simulink model "reaktor"  (R2016a)
settings: Solver=VariableStepAuto  StartTime=0.0  StopTime=300  RelTol=1e-3
values from neighbouring files (symbols this model uses):
  B = 0.0064    [Unit_3.m]    (also in reactor_pocz.m; unit_1.m; unit_4.m)
  C_psi = 13.75 * (10 ^ 6)    (= 13750000)    [Unit_3.m]    (also in reactor_pocz.m; unit_4.m)
  LAMBDA = 10 ^ -5    (= 1e-05)    [Unit_3.m]    (also in reactor_pocz.m; unit_1.m; unit_4.m)
  lambda = 0.1    [Unit_3.m]    (also in reactor_pocz.m; unit_1.m; unit_4.m)
  P_1 = -1.223 * (10 ^ -4)    (= -0.0001223)    [Unit_3.m]    (also in reactor_pocz.m; unit_1.m = -0.0001322; unit_4.m = -0.0001286)
  P_2 = -5.502 * (10 ^ -5)    (= -5.502e-05)    [Unit_3.m]    (also in reactor_pocz.m; unit_1.m = -6.08e-05; unit_4.m = -6.79e-05)
  P_3 = -1.953 * (10 ^ -4)    (= -0.0001953)    [Unit_3.m]    (also in reactor_pocz.m; unit_1.m = -0.000285; unit_4.m = -0.0002887)
  S = 1938.9    [Unit_3.m]    (also in reactor_pocz.m; unit_1.m = 2859; unit_4.m = 2910.3)
settings Model: Creator=Użytkownik  LastModifiedBy=Użytkownik

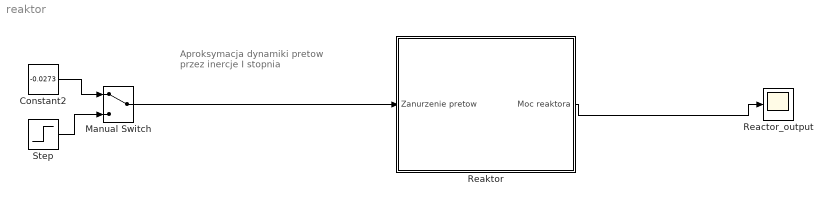
== system reaktor ==
  note: Aproksymacja dynamiki
      | pretow przez inercje I stopnia
  Constant2 : Constant  Value=-0.0273
  Manual Switch : ManualSwitch
  Reactor_output : Scope
  Reaktor : Subsystem
  Step : Step  Time=200  After=10  SampleTime=0
  wires:
  Reaktor/1(Moc reaktora) -> Reactor_output/1
  Manual Switch/1 -> Reaktor/1(Zanurzenie pretow)
  Constant2/1 -> Manual Switch/1
  Step/1 -> Manual Switch/2

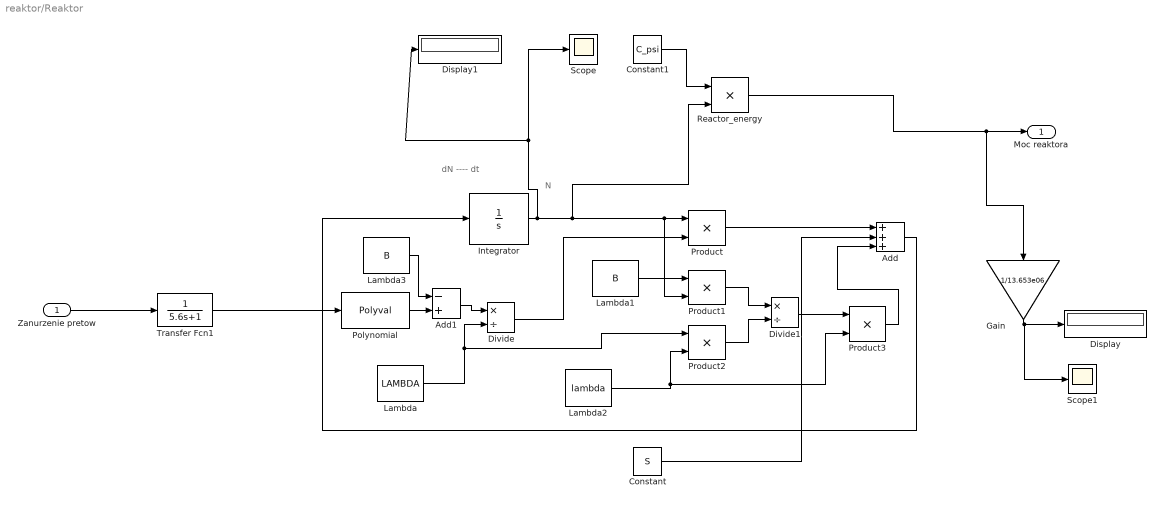
== system reaktor/Reaktor ==
  note: N
  note: dN
      | ----
      | dt
  Zanurzenie pretow : Inport
  Add : Sum  Inputs=+++
  Add1 : Sum  Inputs=-+
  Constant : Constant  Value=S
  Constant1 : Constant  Value=C_psi
  Display : Display
  Display1 : Display
  Divide : Product  Inputs=*/
  Divide1 : Product  Inputs=*/
  Gain : Gain  Gain=1/13.653e06
  Integrator : Integrator
  Lambda : Constant  Value=LAMBDA
  Lambda1 : Constant  Value=B
  Lambda2 : Constant  Value=lambda
  Lambda3 : Constant  Value=B
  Polynomial : Polyval  Coefs=[P_1, P_2, P_3]
  Product{,1..3} (4 alike) : Product
  Reactor_energy : Product
  Scope : Scope
  Scope1 : Scope
  Transfer Fcn1 : TransferFcn  Denominator=[5.6 1]
  Moc reaktora : Outport
  wires:
  Integrator/1 -> Reactor_energy/2, Product1/2, Product/1, Display1/1, Scope/1
  Product/1 -> Add/1
  Constant/1 -> Add/2
  Add/1 -> Integrator/1
  Lambda/1 -> Product2/1, Divide/2
  Divide/1 -> Product/2
  Constant1/1 -> Reactor_energy/1
  Reactor_energy/1 -> Gain/1, Moc reaktora/1
  Lambda1/1 -> Product1/1
  Lambda2/1 -> Product2/2, Product3/2
  Product1/1 -> Divide1/1
  Product2/1 -> Divide1/2
  Divide1/1 -> Product3/1
  Product3/1 -> Add/3
  Lambda3/1 -> Add1/1
  Polynomial/1 -> Add1/2
  Add1/1 -> Divide/1
  Transfer Fcn1/1 -> Polynomial/1
  Zanurzenie pretow/1 -> Transfer Fcn1/1
  Gain/1 -> Scope1/1, Display/1
